simulink model "linearized"  (R2017a)
settings: Solver=VariableStepAuto  StartTime=0.0  StopTime=2000  RelTol=1e-3
undefined symbols (not defined in the file): A, B, C, D, y
settings Model: Creator=WIN10  LastModifiedBy=WIN10

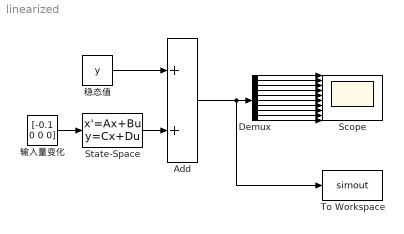
== system linearized ==
  Add : Sum
  Demux : Demux  Outputs=10
  Scope : Scope  NumInputPorts=10
  State-Space : StateSpace  A=A  B=B  C=C  D=D  X0=[0 0 0 0 0 0 0 0 0 0]
  To Workspace : ToWorkspace  VariableName=simout  SaveFormat=Timeseries  SampleTime=-1
  稳态值 : Constant  Value=y
  输入量变化 : Constant  Value=[-0.1 0 0 0]
  wires:
  输入量变化/1 -> State-Space/1
  Demux/1 -> Scope/1
  Demux/2 -> Scope/2
  Demux/3 -> Scope/3
  Demux/4 -> Scope/4
  Demux/5 -> Scope/5
  Demux/6 -> Scope/6
  Demux/7 -> Scope/7
  Demux/8 -> Scope/8
  Demux/9 -> Scope/9
  Demux/10 -> Scope/10
  State-Space/1 -> Add/2
  Add/1 -> To Workspace/1, Demux/1
  稳态值/1 -> Add/1
